simulink model "sf_newtons_cradle"  (Simulink 7.6)
settings: Solver=ode45  SolverMode=SingleTasking  StartTime=0.0  StopTime=5  RelTol=1e-3
settings Model: Creator=The MathWorks Inc.
settings OptimizationCC: BlockReduction=off  BooleanDataType=off  InitFltsAndDblsToZero=on
settings DebuggingCC: SignalResolutionControl=TryResolveAllWithWarning  SolverPrmCheckMsg=none  StrictBusMsg=Warning
settings HardwareCC: TargetUnknown=on
settings SFSimCC: SFSimEnableDebug=off  SFSimOverflowDetection=off  SFSimEcho=off  SimParseCustomCode=off
settings GRTTargetCC: TargetFcnLib=ansi_tfl_tmw_new.mat

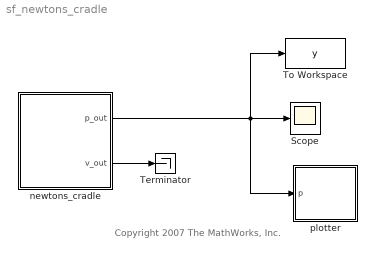
== system sf_newtons_cradle ==
  note: Copyright 2007 The MathWorks, Inc.
  Scope : Scope
      settings: YMin=-0.75  YMax=0.75
  Terminator : Terminator
  To Workspace : ToWorkspace  VariableName=y  SampleTime=-1  SaveFormat=Array
  newtons_cradle : Stateflow chart  TreatAsAtomicUnit=on
  plotter : Stateflow chart  TreatAsAtomicUnit=on
  wires:
  newtons_cradle/1(p_out) -> Scope/1, To Workspace/1, plotter/1(p)
  newtons_cradle/2(v_out) -> Terminator/1

== stateflow chart newtons_cradle ==
  settings: updateMethod=CONTINUOUS  executeAtInitialization=1  initializeOutput=1
  state FreeDynamics
    du:
    p_out = p;
    v_out = v;
    p_dot = v;
    v_dot = -g/l*sin(p);
  state resetPositionsAndVelocities [function]
    (junction 6) -> (junction 11) : {i++;}
    (junction 13) -> (junction 6) [order 2]
    (default) -> (junction 11) : {i=0;}
    (junction 11) -> (junction 12) [order 2]
    (junction 11) -> (junction 13) [order 1] : [i < k-1]
    (junction 13) -> (junction 6) [order 1] : [p[i] < p[i+1]]
        | {
        | // swap positions
        | tmp = p[i];
        | p[i] = p[i+1];
        | p[i+1] = tmp;
        | // swap velocities
        | tmp = v[i];
        | v[i] = v[i+1];
        | v[i+1] = tmp;
        | }
  state collision = isCollisionPossible [function]
    (default) -> (junction 7) : {i=0;}
    (junction 7) -> (junction 8) [order 2] : {
        | collision = 0;
        | }
    (junction 7) -> (junction 9) [order 1] : [i < k-1]
    (junction 9) -> (junction 10) [order 1] : [p[i] < p[i+1]]
        | {
        | collision = 1;
        | }
    (junction 9) -> (junction 7) [order 2] : {i++;}
  (default) -> FreeDynamics : {
      | p = 0;
      | v = 0;
      | p[0] = pi/6;
      | p[1] = pi/6;
      |
      | // uncomment the lines below to see
      | // some interesting behavior
      | // p[k-3] = -pi/6;
      | // p[k-2] = -pi/6;
      | // p[k-1] = -pi/6;
      | // v[0] = 2;
      | }
  FreeDynamics -> FreeDynamics : [isCollisionPossible()]
      | { resetPositionsAndVelocities(); }
  data: i temporary double; tmp temporary double; collision function_output double; i temporary double; p_out output double size=k; v_out output double size=k; g constant double =9.81; l constant double =1; pi constant double =3.141; p local double size=k; v local double size=k; k constant int32 =7
  data p settings: updateMethod=SF_CONTINUOUS_TIME_DATA
  data v settings: updateMethod=SF_CONTINUOUS_TIME_DATA

== stateflow chart plotter ==
  settings: updateMethod=DISCRETE  sampleTime=0.1
  state A
    du:
    ml.sf_newtons_cradle_plotter(p);
  data: p input double
